simulink model "BehPrepUnit"  (R2026a)
settings: Solver=VariableStepAuto
model workspace (MAT data in the model file):
  PrepRate_bph = 100
  PrepTau_s = 60
settings Model: DataDictionary=BehParamsCommon.sldd  ParameterArgumentNames=PrepRate_bph,PrepTau_s  Creator=sarah  LastModifiedBy=sarah

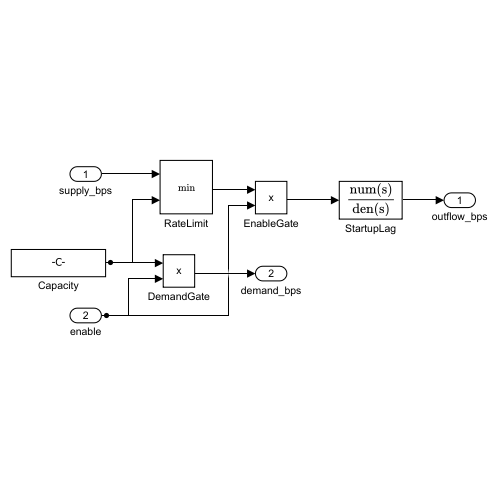
[thumbnail: Simulink's stored preview of the top-level diagram]
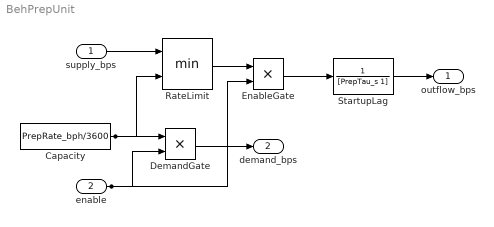
== system BehPrepUnit ==
  supply_bps : Inport
  enable : Inport  Port=2
  Capacity : Constant  Value=PrepRate_bph/3600
  DemandGate : Product
  EnableGate : Product
  RateLimit : MinMax  Inputs=2
  StartupLag : TransferFcn  Denominator=[PrepTau_s 1]
  outflow_bps : Outport
  demand_bps : Outport  Port=2
  wires:
  DemandGate/1 -> demand_bps/1
  supply_bps/1 -> RateLimit/1
  EnableGate/1 -> StartupLag/1
  Capacity/1 -> RateLimit/2, DemandGate/1
  enable/1 -> EnableGate/2, DemandGate/2
  RateLimit/1 -> EnableGate/1
  StartupLag/1 -> outflow_bps/1
